simulink model "samplModel_R2015a_2"  (R2015a)
settings: Solver=FixedStepDiscrete  StartTime=0.0  StopTime=10  RelTol=1e-3
libraries: lib x1
settings Model: Creator=stozaki  LastModifiedBy=stozaki
settings DataIOCC: VisualizeSimOutput=off
settings OptimizationCC: InlineParams=on  OptimizeModelRefInitCode=on  LifeSpan=1
settings DebuggingCC: AlgebraicLoopMsg=error  ParameterDowncastMsg=warning  ParameterOverflowMsg=warning  ParameterUnderflowMsg=warning  FixptConstUnderflowMsg=warning  FixptConstOverflowMsg=warning  FixptConstPrecisionLossMsg=warning  StateNameClashWarn=warning
settings HardwareCC: ProdHWDeviceType=Generic->32-bit Embedded Processor  TargetHWDeviceType=Generic->Custom  ProdEqTarget=off
settings RTWCC: SystemTargetFile=ert.tlc  TemplateMakefile=ert_default_tmf  Description=Embedded Coder  GenerateReport=on  IncludeHyperlinkInReport=on  LaunchReport=on  GenerateCodeMetricsReport=on
settings CodeAppCC: IgnoreCustomStorageClasses=off
settings ERTTargetCC: ParMdlRefBuildCompliant=on  CompOptLevelCompliant=on  ConcurrentExecutionCompliant=on  ERTFirstTimeCompliant=on  SupportContinuousTime=off  SupportVariableSizeSignals=off  ModelStepFunctionPrototypeControlCompliant=on  CPPClassGenCompliant=on  ERTCustomFileTemplate=example_file_process.tlc

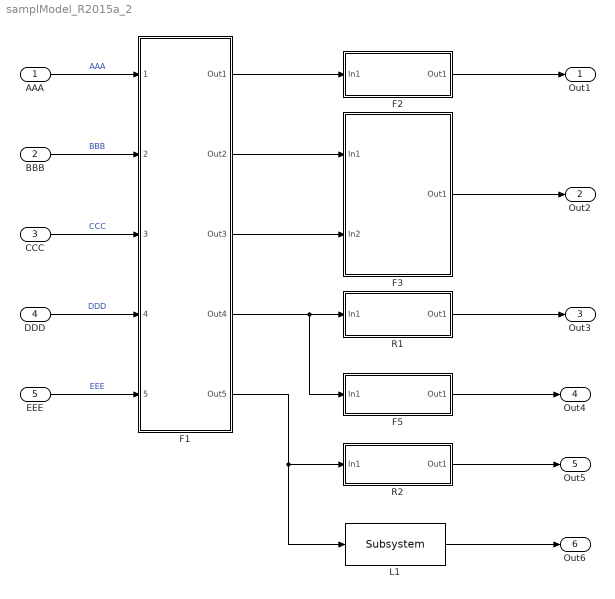
== system samplModel_R2015a_2 ==
  AAA : Inport
  BBB : Inport  Port=2
  CCC : Inport  Port=3
  DDD : Inport  Port=4
  EEE : Inport  Port=5
  F1 : Subsystem  TreatAsAtomicUnit=on
  F2 : Subsystem  TreatAsAtomicUnit=on
  F3 : Subsystem  TreatAsAtomicUnit=on
  F5 : Subsystem  TreatAsAtomicUnit=on
  L1 : lib/Subsystem
  R1 : Subsystem  Description=再利用可能関数  TreatAsAtomicUnit=on
      settings: AttributesFormatString=%<Description>
  R2 : Subsystem  Description=再利用可能関数  TreatAsAtomicUnit=on
      settings: AttributesFormatString=%<Description>
  Out1 : Outport
  Out2 : Outport  Port=2
  Out3 : Outport  Port=3
  Out4 : Outport  Port=4
  Out5 : Outport  Port=5
  Out6 : Outport  Port=6
  wires:
  AAA/1 -> F1/1(1)  "AAA"
  BBB/1 -> F1/2(2)  "BBB"
  CCC/1 -> F1/3(3)  "CCC"
  DDD/1 -> F1/4(4)  "DDD"
  EEE/1 -> F1/5(5)  "EEE"
  F1/1(Out1) -> F2/1(In1)
  F1/2(Out2) -> F3/1(In1)
  F1/3(Out3) -> F3/2(In2)
  F1/4(Out4) -> F5/1(In1), R1/1(In1)
  F1/5(Out5) -> R2/1(In1), L1/1
  F2/1(Out1) -> Out1/1
  F3/1(Out1) -> Out2/1
  R1/1(Out1) -> Out3/1
  F5/1(Out1) -> Out4/1
  R2/1(Out1) -> Out5/1
  L1/1 -> Out6/1

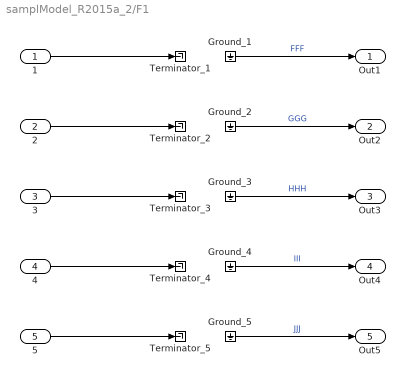
== system samplModel_R2015a_2/F1 ==
  1 : Inport
  2 : Inport  Port=2
  3 : Inport  Port=3
  4 : Inport  Port=4
  5 : Inport  Port=5
  Ground_{1..5} (5 alike) : Ground
  Terminator_{1..5} (5 alike) : Terminator
  Out1 : Outport
  Out2 : Outport  Port=2
  Out3 : Outport  Port=3
  Out4 : Outport  Port=4
  Out5 : Outport  Port=5
  wires:
  1/1 -> Terminator_1/1
  2/1 -> Terminator_2/1
  3/1 -> Terminator_3/1
  4/1 -> Terminator_4/1
  5/1 -> Terminator_5/1
  Ground_1/1 -> Out1/1  "FFF"
  Ground_2/1 -> Out2/1  "GGG"
  Ground_3/1 -> Out3/1  "HHH"
  Ground_4/1 -> Out4/1  "III"
  Ground_5/1 -> Out5/1  "JJJ"

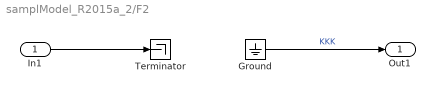
== system samplModel_R2015a_2/F2 ==
  In1 : Inport
  Ground : Ground
  Terminator : Terminator
  Out1 : Outport
  wires:
  Ground/1 -> Out1/1  "KKK"
  In1/1 -> Terminator/1

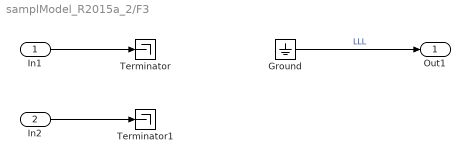
== system samplModel_R2015a_2/F3 ==
  In1 : Inport
  In2 : Inport  Port=2
  Ground : Ground
  Terminator : Terminator
  Terminator1 : Terminator
  Out1 : Outport
  wires:
  Ground/1 -> Out1/1  "LLL"
  In1/1 -> Terminator/1
  In2/1 -> Terminator1/1

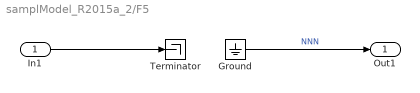
== system samplModel_R2015a_2/F5 ==
  In1 : Inport
  Ground : Ground
  Terminator : Terminator
  Out1 : Outport
  wires:
  Ground/1 -> Out1/1  "NNN"
  In1/1 -> Terminator/1

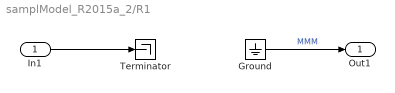
== system samplModel_R2015a_2/R1 ==
  In1 : Inport
  Ground : Ground
  Terminator : Terminator
  Out1 : Outport
  wires:
  Ground/1 -> Out1/1  "MMM"
  In1/1 -> Terminator/1

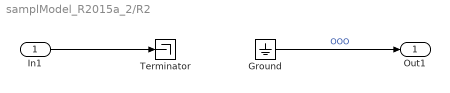
== system samplModel_R2015a_2/R2 ==
  In1 : Inport
  Ground : Ground
  Terminator : Terminator
  Out1 : Outport
  wires:
  Ground/1 -> Out1/1  "OOO"
  In1/1 -> Terminator/1
